simulink model "SMD_system_for_Data_Generation"  (R2023a)
settings: Solver=FixedStepAuto  StartTime=0.0  StopTime=25  FixedStep=0.01  RelTol=1e-3
undefined symbols (not defined in the file or in its folder): DiscIntNeverNeededParam
settings Model: Creator=Z0150218  LastModifiedBy=Z0150218

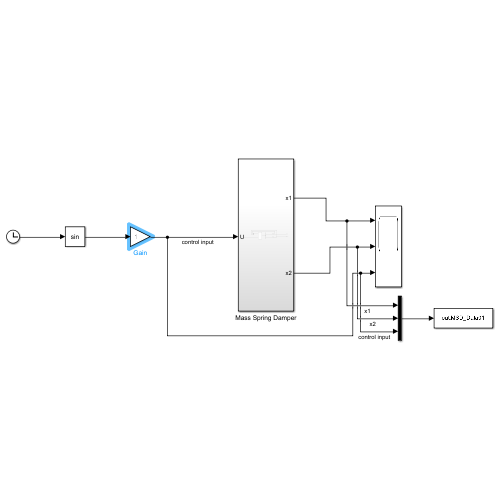
[thumbnail: Simulink's stored preview of the top-level diagram]
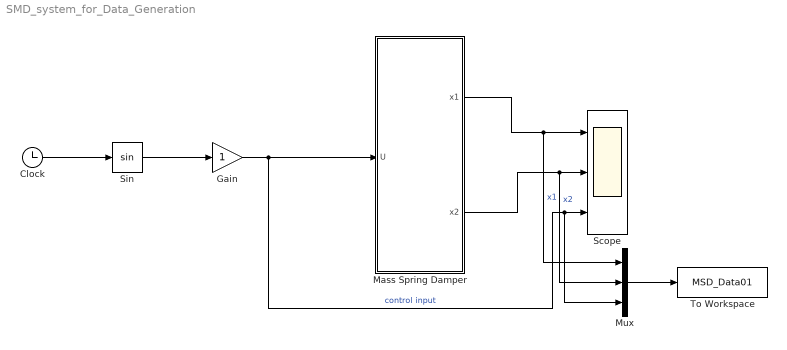
== system SMD_system_for_Data_Generation ==
  Clock : Clock
  Gain : Gain
  Mass Spring Damper : Subsystem
  Mux : Mux  Inputs=3
  Scope : Scope  NumInputPorts=3
  Sin : Trigonometry
  To Workspace : ToWorkspace  VariableName=MSD_Data01  SampleTime=-1
  wires:
  Clock/1 -> Sin/1
  Sin/1 -> Gain/1
  Mass Spring Damper/1(x1) -> Mux/1, Scope/1  "x1"
  Mass Spring Damper/2(x2) -> Mux/2, Scope/2  "x2"
  Gain/1 -> Mux/3, Scope/3, Mass Spring Damper/1(U)  "control input"
  Mux/1 -> To Workspace/1

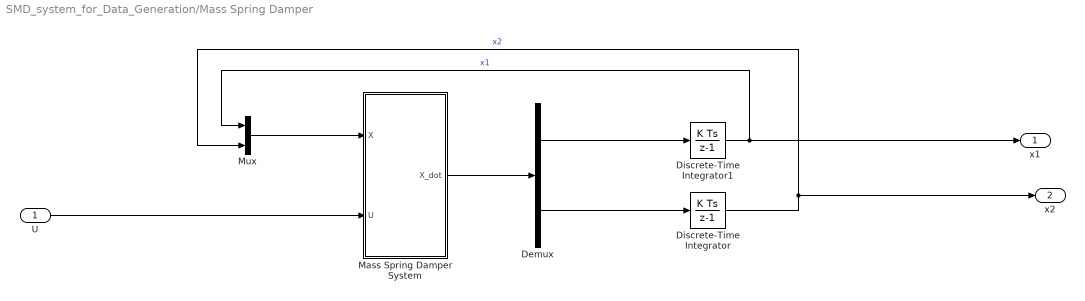
== system SMD_system_for_Data_Generation/Mass Spring Damper ==
  U : Inport
  Demux : Demux  Outputs=2
  Discrete-Time Integrator : DiscreteIntegrator  SampleTime=-1  ICPrevOutput=DiscIntNeverNeededParam  ICPrevScaledInput=DiscIntNeverNeededParam
  Discrete-Time Integrator1 : DiscreteIntegrator  InitialCondition=2.5  SampleTime=-1  ICPrevOutput=DiscIntNeverNeededParam  ICPrevScaledInput=DiscIntNeverNeededParam
  Mass Spring Damper System : MATLAB Function  TreatAsAtomicUnit=on
  Mux : Mux  Inputs=2
  x1 : Outport
  x2 : Outport  Port=2
  wires:
  Discrete-Time Integrator/1 -> Mux/2, x2/1  "x2"
  Discrete-Time Integrator1/1 -> x1/1, Mux/1  "x1"
  Demux/1 -> Discrete-Time Integrator1/1
  Demux/2 -> Discrete-Time Integrator/1
  U/1 -> Mass Spring Damper System/2(U)
  Mass Spring Damper System/1(X_dot) -> Demux/1
  Mux/1 -> Mass Spring Damper System/1(X)

== matlab function SMD_system_for_Data_Generation/Mass Spring Damper/Mass Spring Damper System ==
  data: X input; X_dot output; U input
function X_dot = fcn(X,U)
m = 5;
k = 10;
c = 2;

A = [0 1; -k/m -c/m];
B = [0; 1/m];

X_dot = (A*X)+ (B.*U);

end
